simulink model "basic_PI_model"  (R2024b)
settings: Solver=ode23tb  StartTime=0.0  StopTime=0.4  RelTol=1e-3
InitFcn:
  | pn = 4;
  | Ld = 5.25e-3;
  | Lq = 12e-3;
  | R = 0.958;
  | phi = 0.1827;
  | J = 0.003;
  | B = 0.008;
  | 
  | beta = 50;% speed loop bandwidth rad/s
  | Ba = (beta*J-B)/(1.5*pn*phi);
  | Kpw = beta*J/(1.5*pn*phi);
  | Kiw = beta*Kpw;
  | 
  | tao = min(Ld/R,Lq/R);
  | alpha = 2*pi/tao;
undefined symbols (not defined in the file or in its folder): DiscIntNeverNeededParam
libraries: spsUniversalBridgeLib x1, spsPermanentMagnetSynchronousMachineLib x1, spsSVPWMGenerator2LevelLib x1, spsDCVoltageSourceLib x1, spsabctodq0Lib x1, sps_lib x1

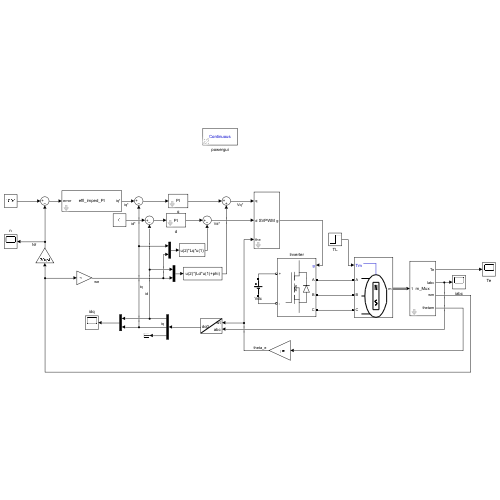
[thumbnail: Simulink's stored preview of the top-level diagram]
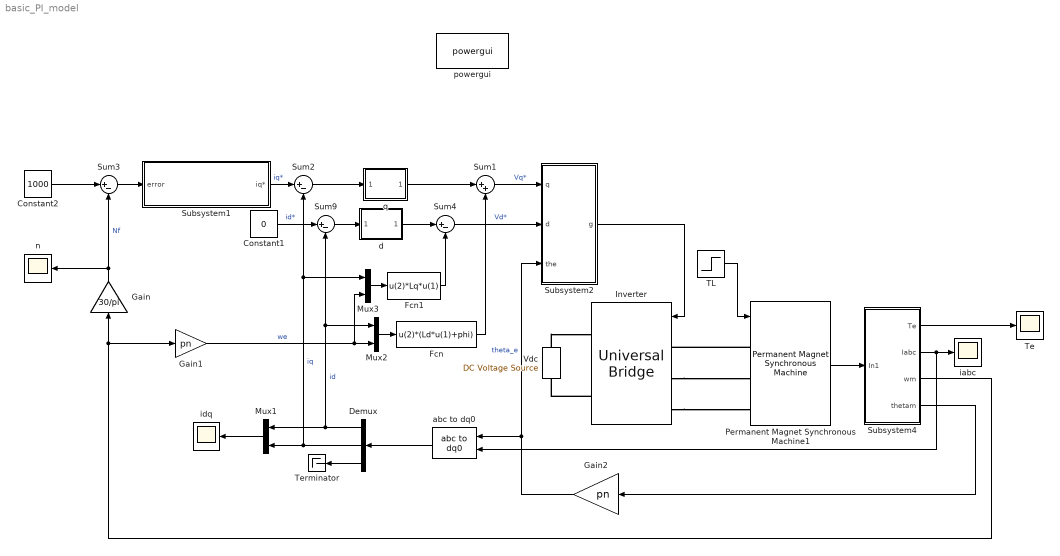
== system basic_PI_model ==
  Constant1 : Constant  Value=0
  Constant2 : Constant  Value=1000
  Demux : Demux  Outputs=3
  Fcn : Fcn  Expr=u(2)*(Ld*u(1)+phi)
  Fcn1 : Fcn  Expr=u(2)*Lq*u(1)
  Gain : Gain  Gain=30/pi
  Gain1 : Gain  Gain=pn
  Gain2 : Gain  Gain=pn
  Inverter : spsUniversalBridgeLib/Universal Bridge  Arms=3  SnubberResistance=1e5  SnubberCapacitance=inf  Device=MOSFET / Diodes  Ron=1e-3  Lon=0  ForwardVoltages="[  0  0  ]"  ForwardVoltage=0  GTOparameters=[ 10e-6 , 20e-6 ]  IGBTparameters=[ 1e-6 , 2e-6 ]  Measurements=None  Measurements_2=None  converterType=Rectifier
  Mux1 : Mux  Inputs=2
  Mux2 : Mux  Inputs=2
  Mux3 : Mux  Inputs=2
  Permanent Magnet Synchronous Machine1 : spsPermanentMagnetSynchronousMachineLib/Permanent Magnet Synchronous Machine  NbPhases=3  FluxDistribution=Sinusoidal  RotorType=Salient-pole  MechanicalLoad=Torque Tm  PresetModel=No  ShowDetailedParameters=on  MeasurementBus=off  Resistance=R  Inductance=8.5e-3  dqInductances=[Ld Lq]  La=0.000395  MachineConstant=Flux linkage established by magnets (V.s)  Flux=phi  VoltageCst=126.966  TorqueCst=1.05  Flat=120  Mechanical=[J B pn 0]  PolePairs=2  InitialConditions=[0,0, 0,0]  InitialConditions5ph=[0 0 0 0 0 0]  RefAngle=Aligned with phase A axis (original Park)  IterativeDiscreteModel=Trapezoidal non iterative  TsBlock=-1  TsPowergui=0
  Subsystem1 : Subsystem  mask{Kpw=Kpw, Kiw=Kiw, Ba=Ba/(30/pi), int_limit=[-30, 30], output_limit=[-30, 30], freq=3e3}
      mask prompts: Kpw "Kp : propotional"; Kiw "Ki : integral"; Ba "Ba : inpedance parameter"; int_limit "integral limitation : [min, max]"; output_limit "output limitation : [min, max]"; freq "frequency [Hz]"
  Subsystem2 : Subsystem  mask{Vdc=311}
  Subsystem4 : Subsystem
  Sum1 : Sum  Inputs=|++
  Sum{2..4,9} (4 alike) : Sum  Inputs=|+-
  TL : Step  Time=0.2  After=10  SampleTime=0
  Te : Scope
  Terminator : Terminator
  Vdc : spsDCVoltageSourceLib/DC Voltage Source  Amplitude=311  Measurements=None
  abc to dq0 : spsabctodq0Lib/abc to dq0  Alignment=Aligned with phase A axis
  d : Subsystem  mask{Kp=alpha*Ld, Ki=alpha*R, int_limit=[-161.6, 161.6], output_limit=[-311*0.9*sqrt(1/3) 311*0.9*sqrt(1/3)], freq=10e3}
      mask prompts: Kp "Kp : propotional"; Ki "Ki : integral"; int_limit "integral limitation : [min, max]"; output_limit "output limitation : [min, max]"; freq "frequency [Hz]"
  iabc : Scope
  idq : Scope
  n : Scope
  powergui : sps_lib/powergui  Priority=1  SimulationMode=Continuous  SampleTime=10e-6  frequency=60  Iterations=50  frequencyindice=0  Pbase=100e6  ErrMax=1e-4  UnitsV=kV  UnitsW=MW  buscounter=0  FunctionMessages=off  echomessages=off  EnableUseOfTLC=off  CurrentSourceSwitches=off  DisableSnubberDevices=off  DisableRonSwitches=off  DisableVfSwitches=off  DisplayEquations=off  AutomaticDiscreteSolvers=off  SolverType=Tustin/Backward Euler (TBE)  Interpol=off  ExternalGateDelay=off  methode=off  Ts=100  x0status=blocks  SPID=on  SwTol=0  HookPort=off  NonlinearTolerance=1e-4  nMaxIteration=100  ContinueOnMaxIteration=off  RestoreLinks=warning  ResistiveCurrentMeasurement=off  Frange=[0:2:500]  Ylog=off  Xlog=on  ShowGrid=off  save=off  variable=ZData  structure=0  ZoomFFT=off  StartTime=0.0  cycles=1  DisplayStyle=1  fundamental=60  FreqAxis=off  MaxFrequency=1000  frequencyindicesteady=1  RmsSteady=1  display=off
  q : Subsystem  mask{Kp=alpha*Lq, Ki=alpha*R, int_limit=[-161.6, 161.6], output_limit=[-311*0.9*sqrt(1/3) 311*0.9*sqrt(1/3)], freq=10e3}
      mask prompts: Kp "Kp : propotional"; Ki "Ki : integral"; int_limit "integral limitation : [min, max]"; output_limit "output limitation : [min, max]"; freq "frequency [Hz]"
  wires:
  Sum1/1 -> Subsystem2/1(q)  "Vq*"
  Fcn1/1 -> Sum4/2
  Constant1/1 -> Sum9/1  "id*"
  Gain/1 -> Sum3/2, n/1  "Nf"
  TL/1 -> Permanent Magnet Synchronous Machine1/1
  Sum4/1 -> Subsystem2/2(d)  "Vd*"
  Permanent Magnet Synchronous Machine1/1 -> Subsystem4/1(In1)
  Demux/1 -> Mux2/1, Sum9/2, Mux1/1  "id"
  Subsystem4/2(Iabc) -> abc to dq0/1, iabc/1
  Subsystem4/1(Te) -> Te/1
  Subsystem4/3(wm) -> Gain1/1, Gain/1
  Subsystem4/4(thetam) -> Gain2/1
  Subsystem2/1(g) -> Inverter/1
  Mux2/1 -> Fcn/1
  Fcn/1 -> Sum1/2
  Gain1/1 -> Mux3/2, Mux2/2  "we"
  Mux3/1 -> Fcn1/1
  Constant2/1 -> Sum3/1
  Sum2/1 -> q/1(input)
  d/1(ouput) -> Sum4/1
  Sum9/1 -> d/1(input)
  q/1(ouput) -> Sum1/1
  Subsystem1/1(iq*) -> Sum2/1  "iq*"
  Sum3/1 -> Subsystem1/1(error)
  abc to dq0/1 -> Demux/1
  Gain2/1 -> Subsystem2/3(the), abc to dq0/2  "theta_e"
  Demux/3 -> Terminator/1
  Demux/2 -> Mux3/1, Sum2/2, Mux1/2  "iq"
  Mux1/1 -> idq/1
  connections:
  Vdc/RConn1 -- Inverter/RConn1
  Permanent Magnet Synchronous Machine1/LConn1 -- Inverter/LConn1
  Inverter/LConn3 -- Permanent Magnet Synchronous Machine1/LConn3
  Inverter/LConn2 -- Permanent Magnet Synchronous Machine1/LConn2
  Inverter/RConn2 -- Vdc/LConn1

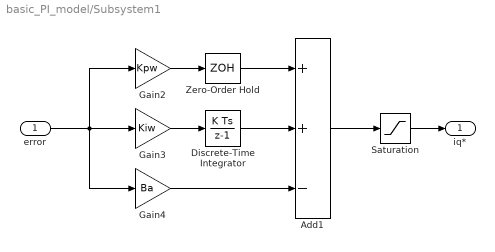
== system basic_PI_model/Subsystem1 ==
  error : Inport
  Add1 : Sum  Inputs=++-
  Discrete-Time Integrator : DiscreteIntegrator  SampleTime=1/freq  LimitOutput=on  UpperSaturationLimit=int_limit(2)  LowerSaturationLimit=int_limit(1)  ICPrevOutput=DiscIntNeverNeededParam  ICPrevScaledInput=DiscIntNeverNeededParam
  Gain2 : Gain  Gain=Kpw
  Gain3 : Gain  Gain=Kiw
  Gain4 : Gain  Gain=Ba
  Saturation : Saturate  UpperLimit=output_limit(2)  LowerLimit=output_limit(1)
  Zero-Order Hold : ZeroOrderHold  SampleTime=1/freq
  iq* : Outport
  wires:
  Add1/1 -> Saturation/1
  Zero-Order Hold/1 -> Add1/1
  Discrete-Time Integrator/1 -> Add1/2
  Gain2/1 -> Zero-Order Hold/1
  Gain3/1 -> Discrete-Time Integrator/1
  Saturation/1 -> iq*/1
  error/1 -> Gain4/1, Gain3/1, Gain2/1
  Gain4/1 -> Add1/3

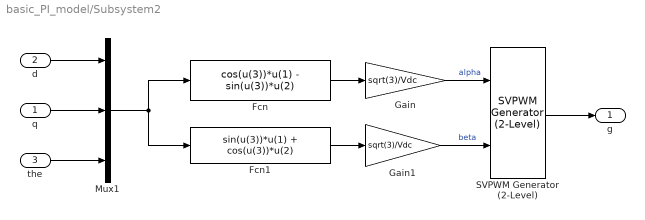
== system basic_PI_model/Subsystem2 ==
  q : Inport
  d : Inport  Port=2
  the : Inport  Port=3
  Fcn : Fcn  Expr=cos(u(3))*u(1) - sin(u(3))*u(2)
  Fcn1 : Fcn  Expr=sin(u(3))*u(1) + cos(u(3))*u(2)
  Gain : Gain  Gain=sqrt(3)/Vdc
  Gain1 : Gain  Gain=sqrt(3)/Vdc
  Mux1 : Mux  Inputs=3
  SVPWM Generator (2-Level) : spsSVPWMGenerator2LevelLib/SVPWM Generator (2-Level)  InputType=alpha-beta components  SwitchingPattern=Pattern #1  Fc=10e3  ParUref=[0.8 -30 50]  Ts=0
  g : Outport
  wires:
  q/1 -> Mux1/2
  Fcn/1 -> Gain/1
  d/1 -> Mux1/1
  Fcn1/1 -> Gain1/1
  SVPWM Generator (2-Level)/1 -> g/1
  Mux1/1 -> Fcn/1, Fcn1/1
  the/1 -> Mux1/3
  Gain/1 -> SVPWM Generator (2-Level)/1  "alpha"
  Gain1/1 -> SVPWM Generator (2-Level)/2  "beta"

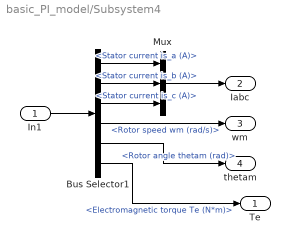
== system basic_PI_model/Subsystem4 ==
  In1 : Inport
  Bus Selector1 : BusSelector  OutputSignals=Stator current is_a (A),Stator current is_b (A),Stator current is_c (A),Rotor speed wm (rad/s),Rotor angle thetam (rad),Electromagnetic torque Te (N*m)
  Mux : Mux  Inputs=3
  Te : Outport
  Iabc : Outport  Port=2
  wm : Outport  Port=3
  thetam : Outport  Port=4
  wires:
  In1/1 -> Bus Selector1/1
  Bus Selector1/1 -> Mux/1  "<Stator current is_a (A)>"
  Bus Selector1/2 -> Mux/2  "<Stator current is_b (A)>"
  Bus Selector1/3 -> Mux/3  "<Stator current is_c (A)>"
  Mux/1 -> Iabc/1
  Bus Selector1/4 -> wm/1  "<Rotor speed wm (rad/s)>"
  Bus Selector1/5 -> thetam/1  "<Rotor angle thetam (rad)>"
  Bus Selector1/6 -> Te/1  "<Electromagnetic torque Te (N*m)>"

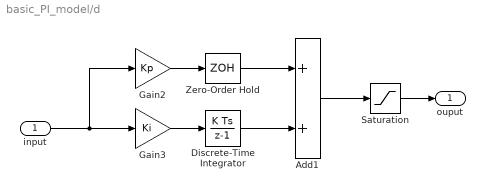
== system basic_PI_model/d ==
  input : Inport
  Add1 : Sum
  Discrete-Time Integrator : DiscreteIntegrator  SampleTime=1/freq  LimitOutput=on  UpperSaturationLimit=int_limit(2)  LowerSaturationLimit=int_limit(1)  ICPrevOutput=DiscIntNeverNeededParam  ICPrevScaledInput=DiscIntNeverNeededParam
  Gain2 : Gain  Gain=Kp
  Gain3 : Gain  Gain=Ki
  Saturation : Saturate  UpperLimit=output_limit(2)  LowerLimit=output_limit(1)
  Zero-Order Hold : ZeroOrderHold  SampleTime=1/freq
  ouput : Outport
  wires:
  Add1/1 -> Saturation/1
  Zero-Order Hold/1 -> Add1/1
  Discrete-Time Integrator/1 -> Add1/2
  Gain2/1 -> Zero-Order Hold/1
  Gain3/1 -> Discrete-Time Integrator/1
  Saturation/1 -> ouput/1
  input/1 -> Gain2/1, Gain3/1

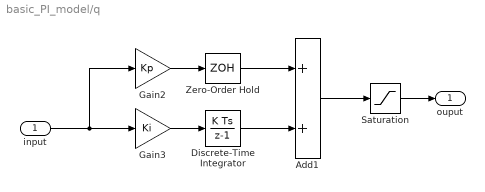
== system basic_PI_model/q ==
  input : Inport
  Add1 : Sum
  Discrete-Time Integrator : DiscreteIntegrator  SampleTime=1/freq  LimitOutput=on  UpperSaturationLimit=int_limit(2)  LowerSaturationLimit=int_limit(1)  ICPrevOutput=DiscIntNeverNeededParam  ICPrevScaledInput=DiscIntNeverNeededParam
  Gain2 : Gain  Gain=Kp
  Gain3 : Gain  Gain=Ki
  Saturation : Saturate  UpperLimit=output_limit(2)  LowerLimit=output_limit(1)
  Zero-Order Hold : ZeroOrderHold  SampleTime=1/freq
  ouput : Outport
  wires:
  Add1/1 -> Saturation/1
  Zero-Order Hold/1 -> Add1/1
  Discrete-Time Integrator/1 -> Add1/2
  Gain2/1 -> Zero-Order Hold/1
  Gain3/1 -> Discrete-Time Integrator/1
  Saturation/1 -> ouput/1
  input/1 -> Gain2/1, Gain3/1
